simulink model "VoltEdge_NITGOA"  (R2024b)
settings: Solver=VariableStepAuto  StartTime=0.0  StopTime=10000  RelTol=1e-3
model workspace (MAT data in the model file):
  ini = 0
undefined symbols (not defined in the file): Ion, Lithium
libraries: spsCurrentMeasurementLib x3, spsVoltageMeasurementLib x3, spsIdealSwitchLib x2, spsBatteryLib x2, simulink_extras x2, dspswit3 x1, spsDCVoltageSourceLib x1, spsGroundLib x1, spsSeriesRLCBranchLib x1, spsMosfetLib x1, simulink x1, sps_lib x1
settings Model: Creator=susha  LastModifiedBy=fliza
settings SolverCC: ZeroCrossAlgorithm=Adaptive
settings DebuggingCC: IgnoredZcDiagnostic=none

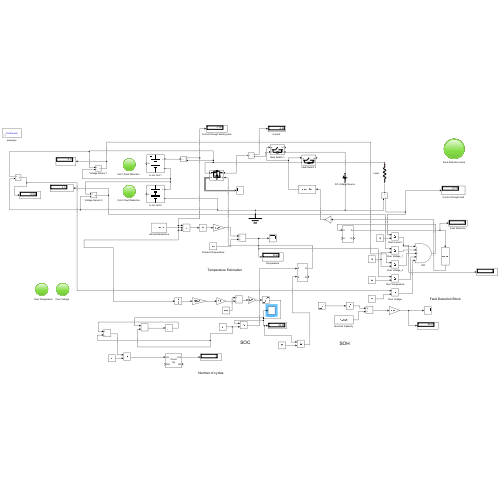
[thumbnail: Simulink's stored preview of the top-level diagram]
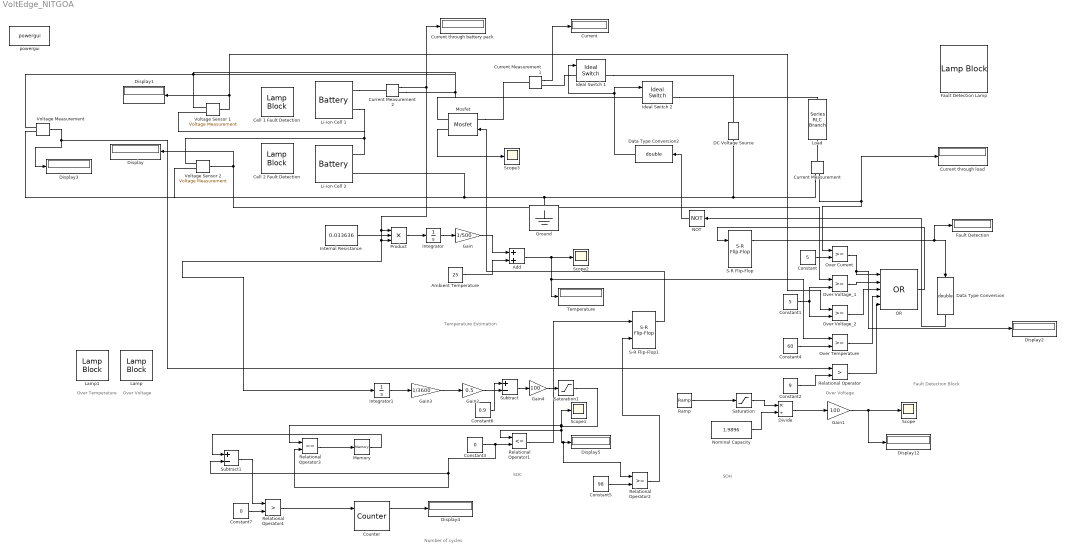
== system VoltEdge_NITGOA ==
  note: Number of cycles
  note: Over Voltage
  note: Over Temperature
  note: Over Voltage
  note: Fault Detection Block
  note: Temperature Estimation
  note: SOC
  note: SOH
  Add : Sum
  Ambient Temperature : Constant  Value=25
  "Cell 1 Fault Detection " : LampBlock  LabelPosition=Hide
  Cell 2 Fault Detection : LampBlock  LabelPosition=Hide
  Constant : Constant  Value=5
  Constant1 : Constant  Value=5
  Constant2 : Constant  Value=9
  Constant3 : Constant  Value=0
  Constant4 : Constant  Value=60
  Constant5 : Constant  Value=98
  Constant6 : Constant  Value=0.9
  Constant7 : Constant  Value=0
  Counter : dspswit3/Counter  Direction=Up  CountEvent=Rising edge  CounterSize=User defined  MaxCount=255  InitialCount=0  Output=Count and Hit  HitValue=32  ResetInput=on  SamplesPerFrame=1  Ts=1  CntDtype=double  HitDtype=Logical
  "Current " : Display
  Current Measurement : spsCurrentMeasurementLib/Current Measurement  PhasorSimulation=off  OutputType=Complex  PSBequivalent=0
  Current Measurement1 : spsCurrentMeasurementLib/Current Measurement  PhasorSimulation=off  OutputType=Complex  PSBequivalent=0
  Current Measurement2 : spsCurrentMeasurementLib/Current Measurement  PhasorSimulation=off  OutputType=Complex  PSBequivalent=0
  Current through battery pack : Display
  Current through load : Display
  DC Voltage Source : spsDCVoltageSourceLib/DC Voltage Source  Amplitude=8.8  Measurements=None
  Data Type Conversion : DataTypeConversion  OutDataTypeStr=double  RndMeth=Floor
  Data Type Conversion2 : DataTypeConversion  OutDataTypeStr=double  RndMeth=Floor
  Display{,1..5,12} (7 alike) : Display
  Divide : Product  Inputs=*/
  Fault Detection : Display
  Fault Detection Lamp : LampBlock  LabelPosition=Hide
  Gain : Gain  Gain=1/500
  Gain1 : Gain  Gain=100
  Gain2 : Gain  Gain=0.5
  Gain3 : Gain  Gain=1/3600
  Gain4 : Gain  Gain=100
  Ground : spsGroundLib/Ground  LConnTagsString=a
  Ideal Switch 1 : spsIdealSwitchLib/Ideal Switch  Ron=0.001  Lon=0  IC=1  Rs=1e5  Cs=inf  Measurements=on
  Ideal Switch 2 : spsIdealSwitchLib/Ideal Switch  Ron=0.001  Lon=0  IC=1  Rs=1e5  Cs=inf  Measurements=on
  Integrator : Integrator
  Integrator1 : Integrator
  Internal Resistance : Constant  Value=0.033636
  Lamp : LampBlock  LabelPosition=Hide
  Lamp1 : LampBlock  LabelPosition=Hide
  Li-ion Cell 1 : spsBatteryLib/Battery  BatType=Lithium-Ion  NomV=3.7  NomQ=2  SOC=90  Batt_Tr=30  PresetModel=on  MaxQ=2  MinV=2.775  FullV=4.3068  Dis_rate=0.86957  R=0.0185  Normal_OP=1.8087  expZone="[3.9974    0.098261]"
  Li-ion Cell 2 : spsBatteryLib/Battery  BatType=Lithium-Ion  NomV=3.7  NomQ=2  SOC=90  Batt_Tr=30  PresetModel=on  MaxQ=2  MinV=2.775  FullV=4.3068  Dis_rate=0.86957  R=0.0185  Normal_OP=1.8087  expZone="[3.9974    0.098261]"
  Load : spsSeriesRLCBranchLib/Series RLC Branch  LConnTagsString=__new0  RConnTagsString=__new0  BranchType=R  Resistance=3  Inductance=0  SetiL0=off  InitialCurrent=0  Capacitance=0  Setx0=off  InitialVoltage=0  Measurements=None
  Memory : Memory
  Mosfet : spsMosfetLib/Mosfet  Ron=0.1  Lon=0  Rd=0.01  Vfd=0  IC=0  Rs=1e5  Cs=inf  Measurements=on
  NOT : Logic  Operator=NOT  IconShape=distinctive  AllPortsSameDT=off  OutDataTypeStr=boolean
  Nominal Capacity : Constant  Value=1.9896
  OR : Logic  Operator=OR  Inputs=5  IconShape=distinctive  AllPortsSameDT=off  OutDataTypeStr=boolean
  "Over Current " : RelationalOperator  OutDataTypeStr=boolean  RndMeth=Simplest  InputSameDT=off
  Over Temperature : RelationalOperator  OutDataTypeStr=boolean  RndMeth=Simplest  InputSameDT=off
  Over Voltage_1 : RelationalOperator  OutDataTypeStr=boolean  RndMeth=Simplest  InputSameDT=off
  Over Voltage_2 : RelationalOperator  OutDataTypeStr=boolean  RndMeth=Simplest  InputSameDT=off
  Product : Product  Inputs=3
  Ramp : simulink/Sources/Ramp  slope=-0.0000829  start=0  InitialOutput=1.9896
  Relational Operator : RelationalOperator  Operator=>  OutDataTypeStr=boolean  RndMeth=Simplest  InputSameDT=off
  Relational Operator1 : RelationalOperator  Operator=<=  OutDataTypeStr=boolean  RndMeth=Simplest  InputSameDT=off
  Relational Operator2 : RelationalOperator  OutDataTypeStr=boolean  RndMeth=Simplest  InputSameDT=off
  Relational Operator3 : RelationalOperator  Operator===  OutDataTypeStr=boolean  RndMeth=Simplest  InputSameDT=off
  Relational Operator4 : RelationalOperator  Operator=>  OutDataTypeStr=boolean  RndMeth=Simplest  InputSameDT=off
  S-R Flip-Flop : simulink_extras/Flip Flops/S-R Flip-Flop  initial_condition=0
  S-R Flip-Flop1 : simulink_extras/Flip Flops/S-R Flip-Flop  initial_condition=0
  Saturation : Saturate  UpperLimit=1.9896  LowerLimit=0
  Saturation1 : Saturate  UpperLimit=100  LowerLimit=0
  Scope{,1..3} (4 alike) : Scope
  Subtract : Sum  Inputs=+-
  Subtract1 : Sum  Inputs=+-
  Temperature : Display
  Voltage Measurement : spsVoltageMeasurementLib/Voltage Measurement  PhasorSimulation=off  OutputType=Complex  PSBequivalent=0
  Voltage Sensor 1 : spsVoltageMeasurementLib/Voltage Measurement  PhasorSimulation=off  OutputType=Complex  PSBequivalent=0
  Voltage Sensor 2 : spsVoltageMeasurementLib/Voltage Measurement  PhasorSimulation=off  OutputType=Complex  PSBequivalent=0
  powergui : sps_lib/powergui  Priority=1  SimulationMode=Continuous  SampleTime=50e-6  frequency=60  Iterations=50  frequencyindice=0  Pbase=100e6  ErrMax=1e-4  UnitsV=kV  UnitsW=MW  buscounter=0  FunctionMessages=off  echomessages=off  EnableUseOfTLC=off  CurrentSourceSwitches=off  DisableSnubberDevices=off  DisableRonSwitches=off  DisableVfSwitches=off  DisplayEquations=off  AutomaticDiscreteSolvers=off  SolverType=Tustin/Backward Euler (TBE)  Interpol=off  ExternalGateDelay=off  methode=off  Ts=100  x0status=blocks  SPID=on  SwTol=0  HookPort=off  NonlinearTolerance=1e-4  nMaxIteration=100  ContinueOnMaxIteration=off  RestoreLinks=warning  ResistiveCurrentMeasurement=off  Frange=[0:2:500]  Ylog=off  Xlog=on  ShowGrid=off  save=off  variable=ZData  structure=0  ZoomFFT=off  StartTime=0.0  cycles=1  DisplayStyle=1  fundamental=60  FreqAxis=off  MaxFrequency=1000  frequencyindicesteady=1  RmsSteady=1  display=off
  wires:
  Constant4/1 -> Over Temperature/2
  Voltage Sensor 1/1 -> Over Voltage_2/1, Display1/1
  OR/1 -> S-R Flip-Flop/1
  Data Type Conversion2/1 -> Ideal Switch 1/1, Ideal Switch 2/1
  Over Voltage_2/1 -> OR/3
  Constant1/1 -> Over Voltage_2/2, Over Voltage_1/2
  Over Temperature/1 -> OR/4
  S-R Flip-Flop/1 -> Fault Detection/1, Data Type Conversion/1
  Internal Resistance/1 -> Product/2
  Current Measurement/1 -> "Over Current "/1, Current through load/1
  NOT/1 -> Data Type Conversion2/1
  Current Measurement1/1 -> "Current "/1
  Data Type Conversion/1 -> NOT/1
  Integrator/1 -> Gain/1
  Product/1 -> Integrator/1
  "Over Current "/1 -> Display2/1, OR/1
  Ambient Temperature/1 -> Add/2
  Gain/1 -> Add/1
  Constant/1 -> "Over Current "/2
  Add/1 -> Scope2/1, Temperature/1, Over Temperature/1
  Over Voltage_1/1 -> OR/2
  Voltage Sensor 2/1 -> Display/1, Over Voltage_1/1
  Ramp/1 -> Saturation/1
  Saturation/1 -> Divide/1
  Nominal Capacity/1 -> Divide/2
  Divide/1 -> Gain1/1
  Gain1/1 -> Scope/1, Display12/1
  Integrator1/1 -> Gain3/1
  Gain2/1 -> Subtract/2
  Constant6/1 -> Subtract/1
  Saturation1/1 -> Relational Operator3/1, Scope1/1, Relational Operator2/1, Display5/1, Relational Operator1/1
  Gain3/1 -> Gain2/1
  Subtract/1 -> Gain4/1
  Gain4/1 -> Saturation1/1
  Voltage Measurement/1 -> Relational Operator/1, Display3/1
  Constant2/1 -> Relational Operator/2
  Relational Operator/1 -> OR/5
  Constant3/1 -> Relational Operator3/2, Subtract1/2, Relational Operator1/2
  Mosfet/1 -> Scope3/1
  Relational Operator1/1 -> S-R Flip-Flop1/1
  Current Measurement2/1 -> Current through battery pack/1, Integrator1/1, Product/3, Product/1
  Constant5/1 -> Relational Operator2/2
  S-R Flip-Flop1/1 -> Mosfet/1
  Relational Operator2/1 -> S-R Flip-Flop1/2
  Relational Operator3/1 -> Memory/1
  Memory/1 -> Subtract1/1
  Subtract1/1 -> Relational Operator4/1
  Constant7/1 -> Relational Operator4/2
  Relational Operator4/1 -> Counter/1
  Counter/1 -> Display4/1
  connections:
  Voltage Sensor 2/LConn1 -- Li-ion Cell 1/LConn2 -- Voltage Sensor 1/LConn2 -- Li-ion Cell 2/LConn1
  Current Measurement/RConn1 -- DC Voltage Source/LConn1 -- Ground/LConn1 -- Voltage Measurement/LConn2 -- Voltage Sensor 2/LConn2 -- Li-ion Cell 2/LConn2
  Ideal Switch 2/LConn1 -- Mosfet/RConn1 -- Current Measurement2/RConn1 -- Voltage Measurement/LConn1 -- Voltage Sensor 1/LConn1
  Ideal Switch 1/LConn1 -- Current Measurement1/RConn1
  Ideal Switch 2/RConn1 -- Load/LConn1
  Li-ion Cell 1/LConn1 -- Current Measurement2/LConn1
  Current Measurement/LConn1 -- Load/RConn1
  Ideal Switch 1/RConn1 -- DC Voltage Source/RConn1
  Mosfet/LConn1 -- Current Measurement1/LConn1
